simulink model "deltaModulation"  (R2023b)
settings: Solver=VariableStepAuto  StartTime=0.0  StopTime=2  RelTol=1e-3
model workspace (MAT data in the model file):
  T = Simulink.Parameter
  T.Value = 0.02
  T.DataType = 'auto'
  T.Complexity = 'real'
  T.Dimensions = [1 1]
libraries: dspsigops x1
settings Model: Creator=sanii  LastModifiedBy=sanii

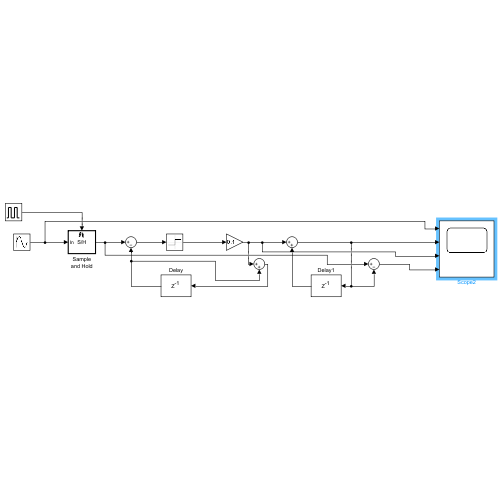
[thumbnail: Simulink's stored preview of the top-level diagram]
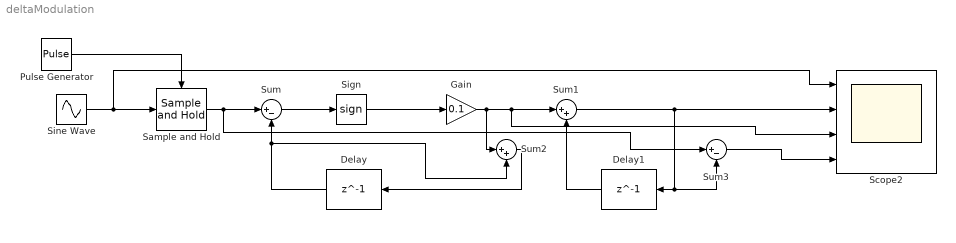
== system deltaModulation ==
  Delay : Delay  DelayLength=1  InitialCondition=0  UseCircularBuffer=on
  Delay1 : Delay  DelayLength=1  InitialCondition=0  UseCircularBuffer=on
  Gain : Gain  Gain=0.1
  Pulse Generator : DiscretePulseGenerator  PulseType=Time based  Period=0.04  PulseWidth=50  VectorParams1D=off
  Sample and Hold : dspsigops/Sample and Hold  trig=Either edge  initCond=0  latchinput=off
  Scope2 : Scope  NumInputPorts=4
  Sign : Signum
  Sine Wave : Sin  Frequency=3  SampleTime=0  VectorParams1D=off
  Sum : Sum  Inputs=|+-
  Sum1 : Sum  Inputs=|++
  Sum2 : Sum  Inputs=|++
  Sum3 : Sum  Inputs=|+-
  wires:
  Pulse Generator/1 -> Sample and Hold/Trigger
  Sample and Hold/1 -> Sum3/1, Sum/1
  Sum/1 -> Sign/1
  Sign/1 -> Gain/1
  Gain/1 -> Sum2/1, Scope2/3, Sum1/1
  Sum2/1 -> Delay/1
  Delay/1 -> Sum2/2, Sum/2
  Delay1/1 -> Sum1/2
  Sum3/1 -> Scope2/4
  Sum1/1 -> Scope2/2, Sum3/2, Delay1/1
  Sine Wave/1 -> Scope2/1, Sample and Hold/1
